simulink model "FanNozzle"  (R2025a)
settings: Solver=VariableStepAuto  StartTime=0.0  StopTime=10.0  RelTol=1e-3
settings Model: Creator=ramch  LastModifiedBy=ramch

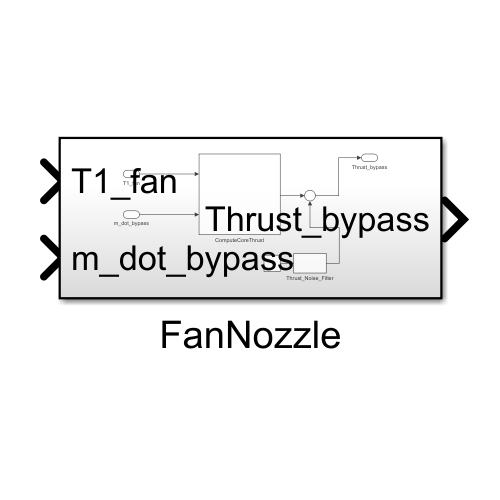
[thumbnail: Simulink's stored preview of the top-level diagram]
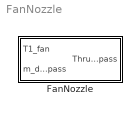
== system FanNozzle ==
  FanNozzle : Subsystem

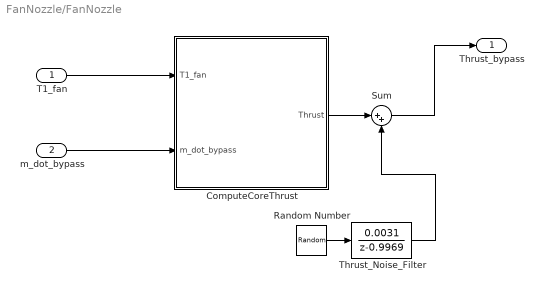
== system FanNozzle/FanNozzle ==
  T1_fan : Inport
  m_dot_bypass : Inport  Port=2
  ComputeCoreThrust : MATLAB Function  TreatAsAtomicUnit=on
  Random Number : RandomNumber  Variance=200  SampleTime=0.001
  Sum : Sum  Inputs=|++
  Thrust_Noise_Filter : DiscreteTransferFcn  Numerator=0.0031  Denominator=1 -0.9969  InitialStates=0.001
  Thrust_bypass : Outport
  wires:
  m_dot_bypass/1 -> ComputeCoreThrust/2(m_dot_bypass)
  ComputeCoreThrust/1(Thrust) -> Sum/1
  Thrust_Noise_Filter/1 -> Sum/2
  Sum/1 -> Thrust_bypass/1
  Random Number/1 -> Thrust_Noise_Filter/1
  T1_fan/1 -> ComputeCoreThrust/1(T1_fan)

== matlab function FanNozzle/ComputeCoreThrust ==
  data: T1_fan input; Thrust output; m_dot_bypass input
function Thrust = ComputeFanThrust(T1_fan, m_dot_bypass)
    cp = 1004;             % J/kg·K (air)
    T_ambient = 288;       % K
    V_ambient = 0;         % m/s, stationary aircraft

    if T1_fan > T_ambient
        V_exit = sqrt(2 * cp * (T1_fan - T_ambient));
    else
        V_exit = 0;
    end

    Thrust = m_dot_bypass * (V_exit - V_ambient);
end
